simulink model "BMS_Software"  (R2021b)
settings: configuration reference "BMS_Sw_CodeGenConfig" (kept outside this file)
undefined symbols (not defined in the file): ts
settings Model: DataDictionary=BMS_Software_DD.sldd  EnableAccessToBaseWorkspace=off  PauseTimes=0  ExtModeTrigDuration=5  Creator=Chirag Patel  LastModifiedBy=lordx
settings ConfigSetRef: SourceName=BMS_Sw_CodeGenConfig

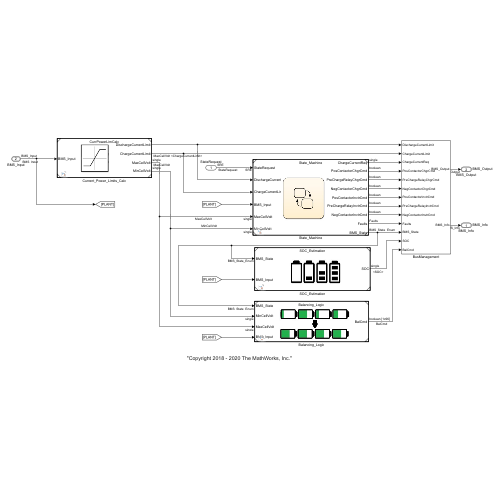
[thumbnail: Simulink's stored preview of the top-level diagram]
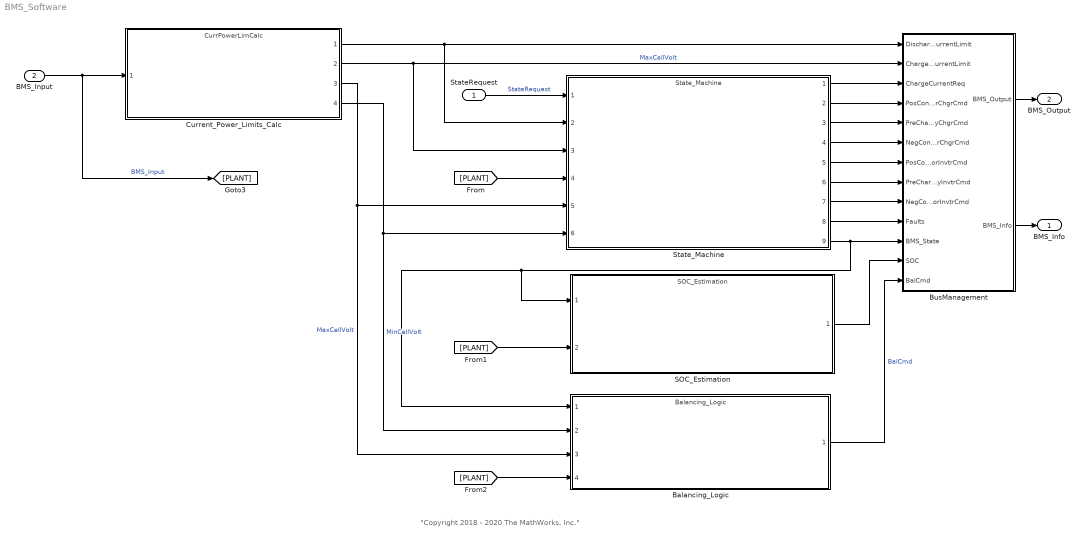
== system BMS_Software ==
  note: "Copyright 2018 - 2020 The MathWorks, Inc."
  StateRequest : Inport  OutDataTypeStr=Enum: SRE  PortDimensions=1  SampleTime=ts
  BMS_Input : Inport  Port=2  OutDataTypeStr=Bus: BMS_Input  BusOutputAsStruct=on
  Balancing_Logic : ModelReference  ModelNameDialog=Balancing_Logic  SimulationMode=Normal  ModelReferenceVersion=3.0
      mask Display: image('Balancing.jpg',[70,5,200,90])
  BusManagement : Subsystem
  Current_Power_Limits_Calc : ModelReference  ModelNameDialog=CurrPowerLimCalc.slx  SimulationMode=Normal  ModelReferenceVersion=3.1
      mask Display: image('CurrentPowerLimit.png',[68,15,80,80])
  SOC_Estimation : ModelReference  ModelNameDialog=SOC_Estimation.slx  SimulationMode=Normal  ModelReferenceVersion=4.1
      mask Display: image('SOC.jpg',[100,15,150,75])
  State_Machine : ModelReference  ModelNameDialog=State_Machine  SimulationMode=Normal  ModelReferenceVersion=3.1
      mask Display: image('StateMachine.jpg',[80,40,130,130])
  BMS_Info : Outport  SignalName=BMS_Info  OutDataTypeStr=Bus: BMS_Info  VectorParamsAs1DForOutWhenUnconnected=off  BusOutputAsStruct=on
  BMS_Output : Outport  Port=2  SignalName=BMS_Output  OutDataTypeStr=Bus: BMS_Output  VectorParamsAs1DForOutWhenUnconnected=off  BusOutputAsStruct=on
  wires:
  BMS_Input/1 -> Current_Power_Limits_Calc/1, [PLANT]  "BMS_Input"
  State_Machine/9 -> SOC_Estimation/1, Balancing_Logic/1, BusManagement/11(BMS_State)
  StateRequest/1 -> State_Machine/1  "StateRequest"
  Current_Power_Limits_Calc/3 -> State_Machine/5, Balancing_Logic/3  "MaxCellVolt"
  Current_Power_Limits_Calc/4 -> Balancing_Logic/2, State_Machine/6  "MinCellVolt"
  [PLANT] -> Balancing_Logic/4
  [PLANT] -> State_Machine/4
  [PLANT] -> SOC_Estimation/2
  State_Machine/1 -> BusManagement/3(ChargeCurrentReq)
  State_Machine/2 -> BusManagement/4(PosContactorChgrCmd)
  State_Machine/3 -> BusManagement/5(PreChargeRelayChgrCmd)
  State_Machine/4 -> BusManagement/6(NegContactorChgrCmd)
  State_Machine/5 -> BusManagement/7(PosContactorInvtrCmd)
  State_Machine/6 -> BusManagement/8(PreChargeRelayInvtrCmd)
  State_Machine/7 -> BusManagement/9(NegContactorInvtrCmd)
  State_Machine/8 -> BusManagement/10(Faults)
  SOC_Estimation/1 -> BusManagement/12(SOC)
  Balancing_Logic/1 -> BusManagement/13(BalCmd)  "BalCmd"
  BusManagement/1(BMS_Output) -> BMS_Output/1
  BusManagement/2(BMS_Info) -> BMS_Info/1
  Current_Power_Limits_Calc/1 -> BusManagement/1(DischargeCurrentLimit), State_Machine/2
  Current_Power_Limits_Calc/2 -> State_Machine/3, BusManagement/2(ChargeCurrentLimit)  "MaxCellVolt"

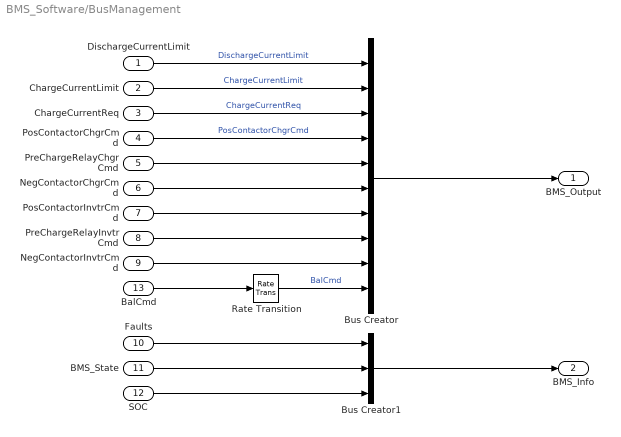
== system BMS_Software/BusManagement ==
  DischargeCurrentLimit : Inport
  ChargeCurrentLimit : Inport  Port=2
  ChargeCurrentReq : Inport  Port=3
  PosContactorChgrCmd : Inport  Port=4
  PreChargeRelayChgrCmd : Inport  Port=5
  NegContactorChgrCmd : Inport  Port=6
  PosContactorInvtrCmd : Inport  Port=7
  PreChargeRelayInvtrCmd : Inport  Port=8
  NegContactorInvtrCmd : Inport  Port=9
  Faults : Inport  Port=10
  BMS_State : Inport  Port=11
  SOC : Inport  Port=12
  BalCmd : Inport  Port=13
  Bus Creator1 : BusCreator  Inputs=3  OutDataTypeStr=Bus: BMS_Info  NonVirtualBus=on
  Bus Creator : BusCreator  Inputs=10  OutDataTypeStr=Bus: BMS_Output  NonVirtualBus=on
  Rate Transition : RateTransition  Integrity=off  Deterministic=off
  BMS_Output : Outport
  BMS_Info : Outport  Port=2  OutDataTypeStr=Bus: BMS_Info
  wires:
  PosContactorInvtrCmd/1 -> Bus Creator/7
  PreChargeRelayChgrCmd/1 -> Bus Creator/5
  PosContactorChgrCmd/1 -> Bus Creator/4  "PosContactorChgrCmd"
  NegContactorInvtrCmd/1 -> Bus Creator/9
  Faults/1 -> Bus Creator1/1
  NegContactorChgrCmd/1 -> Bus Creator/6
  PreChargeRelayInvtrCmd/1 -> Bus Creator/8
  Bus Creator1/1 -> BMS_Info/1
  BalCmd/1 -> Rate Transition/1
  Bus Creator/1 -> BMS_Output/1
  SOC/1 -> Bus Creator1/3
  BMS_State/1 -> Bus Creator1/2
  ChargeCurrentLimit/1 -> Bus Creator/2  "ChargeCurrentLimit"
  DischargeCurrentLimit/1 -> Bus Creator/1  "DischargeCurrentLimit"
  ChargeCurrentReq/1 -> Bus Creator/3  "ChargeCurrentReq"
  Rate Transition/1 -> Bus Creator/10  "BalCmd"
